simulink library "SEN_MTM"  (Simulink 10.2)
settings: Solver=VariableStepAuto  StartTime=0.0  StopTime=10.0  RelTol=1e-3
undefined symbols (not defined in the file): SEN_MTM_par
libraries: simulink x1
settings Model: Creator=dbell44  LastModifiedBy=dbell44

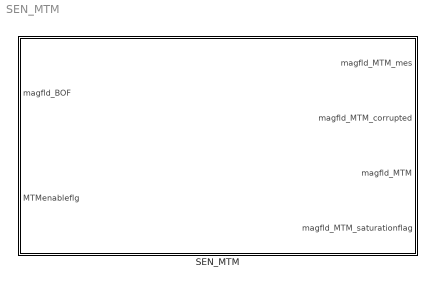
== system SEN_MTM ==
  SEN_MTM : Subsystem

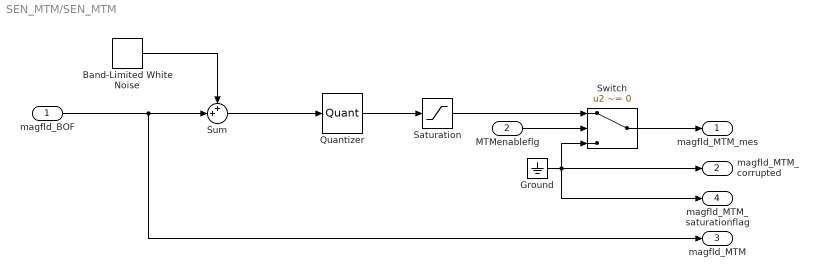
== system SEN_MTM/SEN_MTM ==
  magfld_BOF : Inport
  MTMenableflg : Inport  Port=2
  Band-Limited White Noise : simulink/Sources/Band-Limited White Noise  Cov=SEN_MTM_par.noise_power  Ts=1/SEN_MTM_par.sample_rate  seed=randi([1 243453])
  Ground : Ground
  Quantizer : Quantizer  QuantizationInterval=SEN_MTM_par.sensitivity  LinearizeAsGain=off
  Saturation : Saturate  UpperLimit=SEN_MTM_par.full_scale_range  LowerLimit=-SEN_MTM_par.full_scale_range
  Sum : Sum  Inputs=++|
  Switch : Switch  Criteria=u2 ~= 0
  magfld_MTM_mes : Outport  VectorParamsAs1DForOutWhenUnconnected=off
  magfld_MTM_corrupted : Outport  Port=2  VectorParamsAs1DForOutWhenUnconnected=off
  magfld_MTM : Outport  Port=3  VectorParamsAs1DForOutWhenUnconnected=off
  magfld_MTM_saturationflag : Outport  Port=4  VectorParamsAs1DForOutWhenUnconnected=off
  wires:
  Band-Limited White Noise/1 -> Sum/1
  Sum/1 -> Quantizer/1
  Ground/1 -> magfld_MTM_corrupted/1, magfld_MTM_saturationflag/1, Switch/3
  Quantizer/1 -> Saturation/1
  magfld_BOF/1 -> magfld_MTM/1, Sum/2
  Saturation/1 -> Switch/1
  MTMenableflg/1 -> Switch/2
  Switch/1 -> magfld_MTM_mes/1
